simulink model "Beckeryo"  (Simulink 8.9)
settings: Solver=VariableStepAuto  StartTime=0.0  StopTime=25  FixedStep=0.00001  RelTol=1e-3  EnableMultiTasking=on
settings Model: SuppressorTable=22 serialization::archive 11 0 6 0 0 0 11 0  Creator=joselo  LastModifiedBy=kitsune
settings DataIOCC: SignalLoggingSaveFormat=Dataset
settings DebuggingCC: UnderspecifiedInitializationDetection=Simplified  MergeDetectMultiDrivingBlocksExec=error  FcnCallInpInsideContextMsg=error  StateNameClashWarn=none
settings GRTTargetCC: CombineOutputUpdateFcns=on  GRTInterface=off

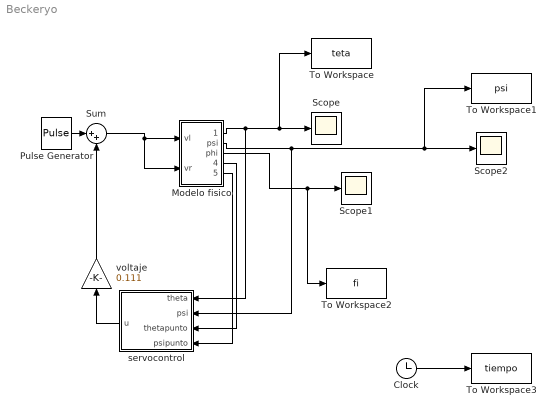
== system Beckeryo ==
  Clock : Clock
  Modelo fisico : Subsystem
  Pulse Generator : DiscretePulseGenerator  PulseType=Time based  TimeSource=Use external signal  Amplitude=100  Period=30  PulseWidth=10
  Scope : Scope
  Scope1 : Scope
  Scope2 : Scope
  Sum : Sum  Inputs=|++
  To Workspace : ToWorkspace  VariableName=teta  SampleTime=-1
  To Workspace1 : ToWorkspace  VariableName=psi  SampleTime=-1
  To Workspace2 : ToWorkspace  VariableName=fi  SampleTime=-1
  To Workspace3 : ToWorkspace  VariableName=tiempo  SampleTime=-1
  servocontrol : Subsystem
  voltaje : Gain  Gain=0.111
  wires:
  Modelo fisico/1(teta) -> servocontrol/1(theta), To Workspace/1, Scope/1
  Modelo fisico/3(phi) -> To Workspace2/1, Scope1/1
  Modelo fisico/2(psi) -> servocontrol/2(psi), To Workspace1/1, Scope2/1
  Pulse Generator/1 -> Sum/1
  voltaje/1 -> Sum/2
  Sum/1 -> Modelo fisico/2(vr), Modelo fisico/1(vl)
  servocontrol/1(u) -> voltaje/1
  Modelo fisico/4(thetadot) -> servocontrol/3(thetapunto)
  Modelo fisico/5(psidot) -> servocontrol/4(psipunto)
  Clock/1 -> To Workspace3/1

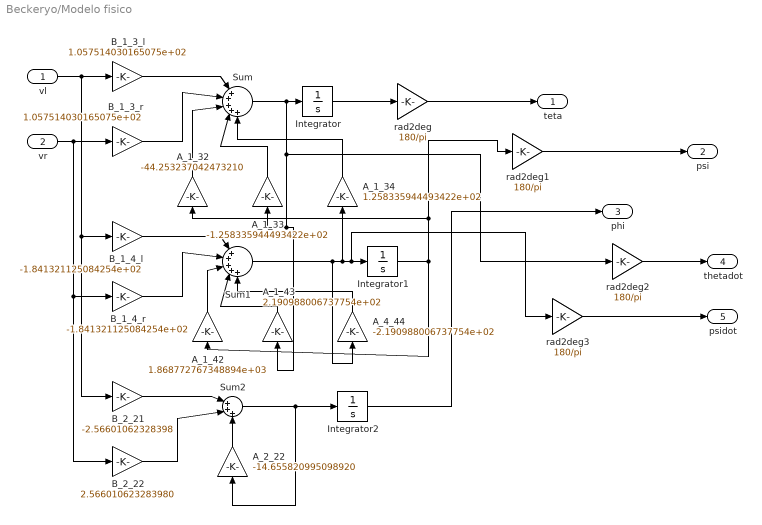
== system Beckeryo/Modelo fisico ==
  vl : Inport
  vr : Inport  Port=2
  A_1_32 : Gain  Gain=-44.253237042473210
  A_1_33 : Gain  Gain=-1.258335944493422e+02
  A_1_34 : Gain  Gain=1.258335944493422e+02
  A_1_42 : Gain  Gain=1.868772767348894e+03
  A_1_43 : Gain  Gain=2.190988006737754e+02
  A_2_22 : Gain  Gain=-14.655820995098920
  A_4_44 : Gain  Gain=-2.190988006737754e+02
  B_1_3_l : Gain  Gain=1.057514030165075e+02
  B_1_3_r : Gain  Gain=1.057514030165075e+02
  B_1_4_l : Gain  Gain=-1.841321125084254e+02
  B_1_4_r : Gain  Gain=-1.841321125084254e+02
  B_2_21 : Gain  Gain=-2.56601062328398
  B_2_22 : Gain  Gain=2.566010623283980
  Integrator : Integrator
  Integrator1 : Integrator
  Integrator2 : Integrator
  Sum : Sum  Inputs=|+++++
  Sum1 : Sum  Inputs=|+++++
  Sum2 : Sum  Inputs=|+++
  rad2deg{,1..3} (4 alike) : Gain  Gain=180/pi
  teta : Outport
  psi : Outport  Port=2
  phi : Outport  Port=3
  thetadot : Outport  Port=4
  psidot : Outport  Port=5
  wires:
  A_2_22/1 -> Sum2/3
  A_1_34/1 -> Sum/5
  B_1_3_r/1 -> Sum/2
  Sum/1 -> rad2deg2/1, A_1_33/1, A_1_43/1, Integrator/1
  Sum1/1 -> A_4_44/1, A_1_34/1, rad2deg3/1, Integrator1/1
  A_1_33/1 -> Sum/4
  B_1_4_r/1 -> Sum1/2
  A_1_32/1 -> Sum/3
  A_4_44/1 -> Sum1/5
  A_1_43/1 -> Sum1/4
  A_1_42/1 -> Sum1/3
  B_2_21/1 -> Sum2/1
  B_1_4_l/1 -> Sum1/1
  Integrator2/1 -> phi/1
  B_1_3_l/1 -> Sum/1
  vl/1 -> B_1_3_l/1, B_2_21/1, B_1_4_l/1
  vr/1 -> B_2_22/1, B_1_4_r/1, B_1_3_r/1
  Sum2/1 -> Integrator2/1, A_2_22/1
  Integrator1/1 -> A_1_42/1, rad2deg1/1, A_1_32/1
  B_2_22/1 -> Sum2/2
  Integrator/1 -> rad2deg/1
  rad2deg/1 -> teta/1
  rad2deg1/1 -> psi/1
  rad2deg2/1 -> thetadot/1
  rad2deg3/1 -> psidot/1

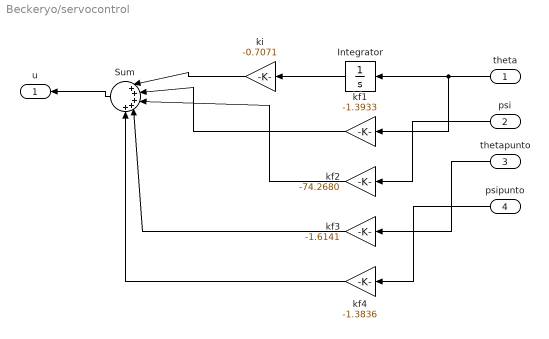
== system Beckeryo/servocontrol ==
  theta : Inport
  psi : Inport  Port=2
  thetapunto : Inport  Port=3
  psipunto : Inport  Port=4
  Integrator : Integrator
  Sum : Sum  Inputs=|+++++
  kf1 : Gain  Gain=-1.3933
  kf2 : Gain  Gain=-74.2680
  kf3 : Gain  Gain=-1.6141
  kf4 : Gain  Gain=-1.3836
  ki : Gain  Gain=-0.7071
  u : Outport
  wires:
  Sum/1 -> u/1
  theta/1 -> kf1/1, Integrator/1
  Integrator/1 -> ki/1
  ki/1 -> Sum/1
  psi/1 -> kf2/1
  thetapunto/1 -> kf3/1
  psipunto/1 -> kf4/1
  kf1/1 -> Sum/2
  kf2/1 -> Sum/3
  kf3/1 -> Sum/4
  kf4/1 -> Sum/5
